simulink model "compressor_linearized"  (Simulink 7.4)
settings: Solver=ode45  StartTime=0.0  StopTime=85  RelTol=1e-3
values from neighbouring files (symbols this model uses):
  P_D = x(end)    [comp_rig_parallel_linearized.m]    (also in comp_rig_tank.m = x(1); get_tank_deriv.m = x(1); setup.m = 0.954; test_linearization.m = P_D_init + delta_x(end,i))
  Ts = 0.05    [const_sim.m]
  uoff1 = [0.304, 0.405, 0.393, 0]'    [const_sim.m]
  uoff2 = [0.304, 0.405, 0.393, 0]'    [const_sim.m]
  x_init_lin = [0.899; 1.126; 0.15; 440; 0]    [comp_rig_parallel_linearized.m]
libraries: dspsrcs4 x3
settings Model: Creator=chkajon  LastModifiedBy=chkajon

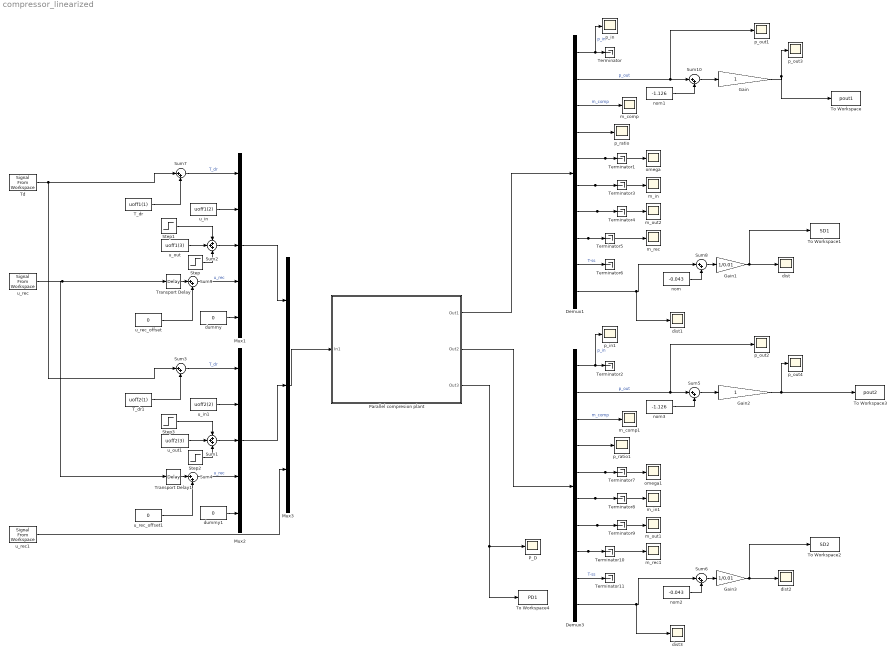
== system compressor_linearized ==
  Demux1 : Demux  Outputs=10
  Demux3 : Demux  Outputs=10
  Gain : Gain
  Gain1 : Gain  Gain=1/0.01
  Gain2 : Gain
  Gain3 : Gain  Gain=1/0.01
  Mux1 : Mux  Inputs=5
  Mux2 : Mux  Inputs=5
  Mux3 : Mux  Inputs=3
  P_D : Scope
      settings: TimeRange=100  YMin=0.03  YMax=0.075  SaveName=ScopeData18
  Parallel compresion plant : Subsystem
      mask Display: image(imread('comp_plant.jpg'))
  Step : Step  Time=50  After=0  SampleTime=0
  Step1 : Step  Time=100  After=0  SampleTime=0
  Step2 : Step  Time=50  After=0  SampleTime=0
  Step3 : Step  Time=100  After=0  SampleTime=0
  Sum1 : Sum  Inputs=+++
  Sum{3..10} (8 alike) : Sum  Inputs=|++
  Sum2 : Sum  Inputs=+++
  T_dr : Constant  Value=uoff1(1)
  T_dr1 : Constant  Value=uoff2(1)
  Td : dspsrcs4/Signal From Workspace  SystemSampleTime=-1  X=Td  Ts=Ts  nsamps=1  OutputAfterFinalValue=Holding final value  ignoreOrWarnInputAndFrameLengths=off
  Terminator{,1..11} (12 alike) : Terminator
  To Workspace : ToWorkspace  VariableName=pout1  SampleTime=-1  SaveFormat=Structure With Time
  To Workspace1 : ToWorkspace  VariableName=SD1  SampleTime=-1  SaveFormat=Structure With Time
  To Workspace2 : ToWorkspace  VariableName=SD2  SampleTime=-1  SaveFormat=Structure With Time
  To Workspace3 : ToWorkspace  VariableName=pout2  SampleTime=-1  SaveFormat=Structure With Time
  To Workspace4 : ToWorkspace  VariableName=PD1  SampleTime=-1  SaveFormat=Structure With Time
  Transport Delay : TransportDelay  DelayTime=1.0
  Transport Delay1 : TransportDelay  DelayTime=1.0
  dist{,1..3} (4 alike) : Scope
      dist settings: YMin=-11  YMax=2
      dist1 settings: TimeRange=100  YMin=0.03  YMax=0.075
      dist2 settings: YMin=-11  YMax=2  SaveName=ScopeData9
      dist3 settings: TimeRange=100  YMin=0.03  YMax=0.075  SaveName=ScopeData10
  dummy : Constant  Value=0
  dummy1 : Constant  Value=0
  m_comp : Scope
      settings: TimeRange=100  YMin=0.5  YMax=0.825  SaveName=m_comp  DataFormat=Array
  m_comp1 : Scope
      settings: TimeRange=100  YMin=0.5  YMax=0.825  SaveName=m_comp1  DataFormat=Array
  m_in : Scope
      settings: TimeRange=100  YMin=100.8  YMax=100.975  SaveName=ScopeData2
  m_in1 : Scope
      settings: TimeRange=100  YMin=100.8  YMax=100.975  SaveName=ScopeData11
  m_out1 : Scope
      settings: TimeRange=100  YMin=100.8  YMax=100.975  SaveName=ScopeData12
  m_out2 : Scope
      settings: TimeRange=100  YMin=100.8  YMax=100.975  SaveName=ScopeData3
  m_rec : Scope
      settings: TimeRange=100  YMin=100.8  YMax=100.975  SaveName=ScopeData4
  m_rec1 : Scope
      settings: TimeRange=100  YMin=100.8  YMax=100.975  SaveName=ScopeData13
  nom : Constant  Value=-0.043
  nom1 : Constant  Value=-1.126
  nom2 : Constant  Value=-0.043
  nom3 : Constant  Value=-1.126
  omega : Scope
      settings: TimeRange=100  YMin=200  YMax=700  SaveName=ScopeData5
  omega1 : Scope
      settings: TimeRange=100  YMin=200  YMax=700  SaveName=ScopeData14
  p_in : Scope
      settings: TimeRange=100  YMin=0.895197  YMax=0.895225  SaveName=ScopeData6
  p_in1 : Scope
      settings: TimeRange=100  YMin=0.895197  YMax=0.895225  SaveName=ScopeData15
  p_out{1..4} (4 alike) : Scope
      p_out1 settings: TimeRange=100  YMin=100.8  YMax=100.975  SaveName=ScopeData7
      p_out2 settings: TimeRange=100  YMin=100.8  YMax=100.975  SaveName=ScopeData16
      p_out3 settings: TimeRange=100  YMin=-2.5  YMax=40  SaveName=ScopeData8
      p_out4 settings: TimeRange=100  YMin=-2.5  YMax=40  SaveName=ScopeData17
  p_ratio : Scope
      settings: TimeRange=100  YMin=0.5  YMax=0.825  SaveName=p_ratio  DataFormat=Array
  p_ratio1 : Scope
      settings: TimeRange=100  YMin=0.5  YMax=0.825  SaveName=p_ratio1  DataFormat=Array
  u_in : Constant  Value=uoff1(2)
  u_in1 : Constant  Value=uoff2(2)
  u_out : Constant  Value=uoff1(3)
  u_out1 : Constant  Value=uoff2(3)
  u_rec : dspsrcs4/Signal From Workspace  SystemSampleTime=-1  X=u_rec  Ts=Ts  nsamps=1  OutputAfterFinalValue=Holding final value  ignoreOrWarnInputAndFrameLengths=off
  u_rec1 : dspsrcs4/Signal From Workspace  SystemSampleTime=-1  X=u_d  Ts=Ts  nsamps=1  OutputAfterFinalValue=Holding final value  ignoreOrWarnInputAndFrameLengths=off
  u_rec_offset : Constant  Value=0
  u_rec_offset1 : Constant  Value=0
  wires:
  Sum2/1 -> Mux1/3
  Step/1 -> Sum2/3
  Transport Delay/1 -> Sum9/1
  dummy/1 -> Mux1/5
  Td/1 -> Sum7/1, Sum3/1
  u_rec_offset/1 -> Sum9/2
  T_dr/1 -> Sum7/2
  Sum9/1 -> Mux1/4  "u_rec"
  Sum7/1 -> Mux1/1  "T_dr"
  u_rec/1 -> Transport Delay/1, Transport Delay1/1
  u_out/1 -> Sum2/2
  u_in/1 -> Mux1/2
  Step1/1 -> Sum2/1
  Sum1/1 -> Mux2/3
  Step2/1 -> Sum1/3
  Transport Delay1/1 -> Sum4/1
  dummy1/1 -> Mux2/5
  u_rec_offset1/1 -> Sum4/2
  T_dr1/1 -> Sum3/2
  Sum4/1 -> Mux2/4  "u_rec"
  Sum3/1 -> Mux2/1  "T_dr"
  u_out1/1 -> Sum1/2
  u_in1/1 -> Mux2/2
  Step3/1 -> Sum1/1
  Mux1/1 -> Mux3/1
  Mux2/1 -> Mux3/2
  Mux3/1 -> Parallel compresion plant/1(In1)
  Demux1/9 -> Terminator6/1  "T-ss"
  Demux1/10 -> Sum8/1, dist1/1
  Gain1/1 -> dist/1, To Workspace1/1
  Gain/1 -> p_out3/1, To Workspace/1
  nom1/1 -> Sum10/2
  Sum10/1 -> Gain/1
  Demux1/4 -> p_ratio/1
  Demux1/5 -> Terminator1/1, omega/1
  Demux1/1 -> Terminator/1, p_in/1  "p_in"
  Demux1/2 -> Sum10/1, p_out1/1  "p_out"
  Sum8/1 -> Gain1/1
  nom/1 -> Sum8/2
  Demux1/7 -> Terminator4/1, m_out2/1
  Demux1/8 -> Terminator5/1, m_rec/1
  Demux1/6 -> Terminator3/1, m_in/1
  Demux1/3 -> m_comp/1  "m_comp"
  Demux3/9 -> Terminator11/1  "T-ss"
  Demux3/10 -> dist3/1, Sum6/1
  Gain3/1 -> dist2/1, To Workspace2/1
  Gain2/1 -> p_out4/1, To Workspace3/1
  nom3/1 -> Sum5/2
  Sum5/1 -> Gain2/1
  Demux3/4 -> p_ratio1/1
  Demux3/5 -> omega1/1, Terminator7/1
  Demux3/1 -> p_in1/1, Terminator2/1  "p_in"
  Demux3/2 -> p_out2/1, Sum5/1  "p_out"
  Sum6/1 -> Gain3/1
  nom2/1 -> Sum6/2
  Demux3/7 -> Terminator9/1, m_out1/1
  Demux3/8 -> m_rec1/1, Terminator10/1
  Demux3/6 -> m_in1/1, Terminator8/1
  Demux3/3 -> m_comp1/1  "m_comp"
  Parallel compresion plant/1(Out1) -> Demux1/1
  Parallel compresion plant/2(Out2) -> Demux3/1
  Parallel compresion plant/3(Out3) -> P_D/1, To Workspace4/1
  u_rec1/1 -> Mux3/3

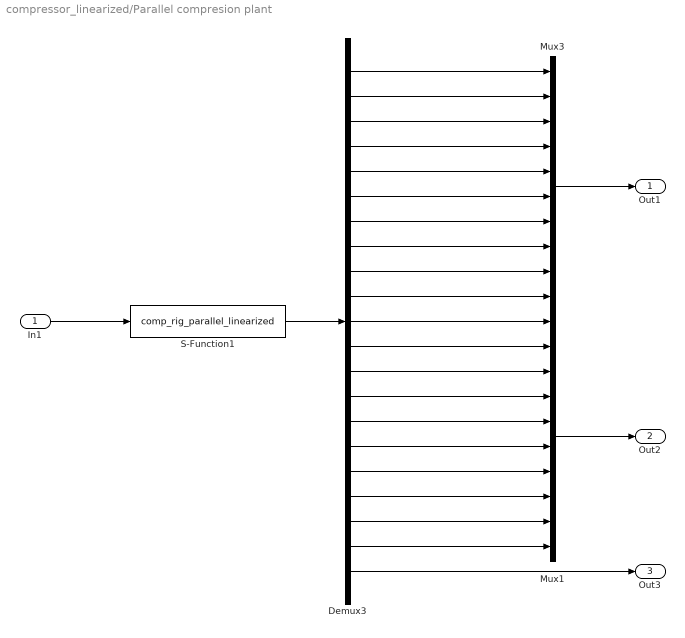
== system compressor_linearized/Parallel compresion plant ==
  In1 : Inport
  Demux3 : Demux  Outputs=21
  Mux1 : Mux  Inputs=10
  Mux3 : Mux  Inputs=10
  S-Function1 : S-Function  FunctionName=comp_rig_parallel_linearized  Parameters=[], [x_init_lin; x_init_lin; P_D]  EnableBusSupport=off
  Out1 : Outport
  Out2 : Outport  Port=2
  Out3 : Outport  Port=3
  wires:
  In1/1 -> S-Function1/1
  Demux3/1 -> Mux3/1
  Demux3/2 -> Mux3/2
  Demux3/3 -> Mux3/3
  Demux3/4 -> Mux3/4
  Demux3/5 -> Mux3/5
  Demux3/6 -> Mux3/6
  Demux3/7 -> Mux3/7
  Demux3/8 -> Mux3/8
  Demux3/9 -> Mux3/9
  Demux3/10 -> Mux3/10
  Demux3/11 -> Mux1/1
  Demux3/12 -> Mux1/2
  Demux3/13 -> Mux1/3
  Demux3/14 -> Mux1/4
  Demux3/15 -> Mux1/5
  Demux3/16 -> Mux1/6
  Demux3/17 -> Mux1/7
  Demux3/18 -> Mux1/8
  Demux3/19 -> Mux1/9
  Demux3/20 -> Mux1/10
  Demux3/21 -> Out3/1
  Mux1/1 -> Out2/1
  Mux3/1 -> Out1/1
  S-Function1/1 -> Demux3/1
